simulink library "csc_cac_coarse_acs_cntrl_mtv_lib"  (R2014b)
settings: Solver=ode45  StartTime=0.0  StopTime=10.0  RelTol=1e-3
values from neighbouring files (symbols this model uses):
  attitude_limit = 0.1745    [csu_waypoint_hover_guidance_init.m]
  fsw_dt = 0.1    [csc_est_state_estimation_test.m]    (also in csci_fsw_mtv_init.m)
  kd_attitude = 5.3    [csu_waypoint_hover_guidance_init.m]
  ki_attitude = 15    [csu_waypoint_hover_guidance_init.m]
  kp_attitude = 14.2    [csu_waypoint_hover_guidance_init.m]
  psp_coarse_acs_thrust = 25.5773    [csu_psp_propulstion_system_parameters_mtv_init.m]
  psp_thruster10_orientation = [0.259,0,0.966]    [csu_psp_propulstion_system_parameters_mtv_init.m]
  psp_thruster10_position = [-0.0699,-0.6668,-0.22]    [csu_psp_propulstion_system_parameters_mtv_init.m]
  psp_thruster11_orientation = [0,0,1]    [csu_psp_propulstion_system_parameters_mtv_init.m]
  psp_thruster11_position = [0,-0.6668,-0.22]    [csu_psp_propulstion_system_parameters_mtv_init.m]
  psp_thruster12_orientation = [-0.259,0,0.966]    [csu_psp_propulstion_system_parameters_mtv_init.m]
  psp_thruster12_position = [0.0699,-0.6668,-0.22]    [csu_psp_propulstion_system_parameters_mtv_init.m]
  psp_thruster1_orientation = [0,0.259,0.966]    [csu_psp_propulstion_system_parameters_mtv_init.m]
  psp_thruster1_position = [0.6668,-0.0699,-0.22]    [csu_psp_propulstion_system_parameters_mtv_init.m]
  psp_thruster2_orientation = [0,0,1]    [csu_psp_propulstion_system_parameters_mtv_init.m]
  psp_thruster2_position = [0.6668,0,-0.22]    [csu_psp_propulstion_system_parameters_mtv_init.m]
  psp_thruster3_orientation = [0,-0.259,0.966]    [csu_psp_propulstion_system_parameters_mtv_init.m]
  psp_thruster3_position = [0.6668,0.0699,-0.22]    [csu_psp_propulstion_system_parameters_mtv_init.m]
  psp_thruster4_orientation = [-0.259,0,0.966]    [csu_psp_propulstion_system_parameters_mtv_init.m]
  psp_thruster4_position = [0.0699,0.6668,-0.22]    [csu_psp_propulstion_system_parameters_mtv_init.m]
  psp_thruster5_orientation = [0,0,1]    [csu_psp_propulstion_system_parameters_mtv_init.m]
  psp_thruster5_position = [0,0.6668,-0.22]    [csu_psp_propulstion_system_parameters_mtv_init.m]
  psp_thruster6_orientation = [0.259,0,0.966]    [csu_psp_propulstion_system_parameters_mtv_init.m]
  psp_thruster6_position = [-0.0699,0.6668,-0.22]    [csu_psp_propulstion_system_parameters_mtv_init.m]
  psp_thruster7_orientation = [0,-0.259,0.966]    [csu_psp_propulstion_system_parameters_mtv_init.m]
  psp_thruster7_position = [-0.6668,0.0699,-0.22]    [csu_psp_propulstion_system_parameters_mtv_init.m]
  psp_thruster8_orientation = [0,0,1]    [csu_psp_propulstion_system_parameters_mtv_init.m]
  psp_thruster8_position = [-0.6668,0,-0.22]    [csu_psp_propulstion_system_parameters_mtv_init.m]
  psp_thruster9_orientation = [0,0.259,0.966]    [csu_psp_propulstion_system_parameters_mtv_init.m]
  psp_thruster9_position = [-0.6668,-0.0699,-0.22]    [csu_psp_propulstion_system_parameters_mtv_init.m]
undefined symbols (not defined in the file or in its folder): coarse_thr_on_bias, emp_cgx_location_fillfrac_100, emp_cgy_location_fillfrac_100, emp_cgz_location_fillfrac_100, emp_inertia_wet_dry, emp_mass_wet_dry, force_1_2_3_7_8_9, force_1_to_12, force_2_8, force_4_5_6_10_11_12, force_5_11, Thr2TqF
libraries: simulink x17, vrlib x12, util_quat_lib x2, util_mass_prop_lib x1
settings Model: Creator=tgorton  LastModifiedBy=tgorton

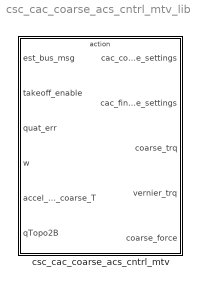
== system csc_cac_coarse_acs_cntrl_mtv_lib ==
  csc_cac_coarse_acs_cntrl_mtv : Subsystem

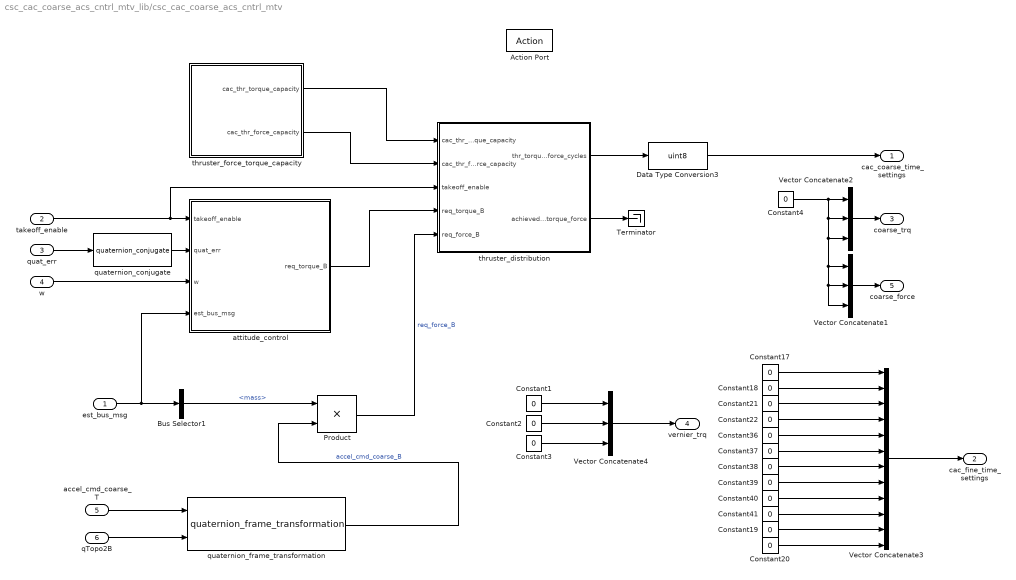
== system csc_cac_coarse_acs_cntrl_mtv_lib/csc_cac_coarse_acs_cntrl_mtv ==
  est_bus_msg : Inport
  takeoff_enable : Inport  Port=2
  quat_err : Inport  Port=3
  w : Inport  Port=4
  accel_cmd_coarse_T : Inport  Port=5
  qTopo2B : Inport  Port=6
  Action Port : ActionPort
  Bus Selector1 : BusSelector  OutputSignals=mass
  Constant{1..4} (4 alike) : Constant  Value=0  OutDataTypeStr=int8
  Constant{17..22,36..41} (12 alike) : Constant  Value=0  OutDataTypeStr=uint8
  Data Type Conversion3 : DataTypeConversion  OutDataTypeStr=uint8
  Product : Product
  Terminator : Terminator
  Vector Concatenate1 : Concatenate  NumInputs=3
  Vector Concatenate2 : Concatenate  NumInputs=3
  Vector Concatenate3 : Concatenate  NumInputs=12
  Vector Concatenate4 : Concatenate  NumInputs=3
  attitude_control : Subsystem
  quaternion_conjugate : util_quat_lib/quaternion_conjugate  SystemSampleTime=-1
  quaternion_frame_transformation : util_quat_lib/quaternion_frame_transformation  SystemSampleTime=-1
  thruster_distribution : Subsystem
  "thruster_force_torque_capacity " : Subsystem
  cac_coarse_time_settings : Outport
  cac_fine_time_settings : Outport  Port=2
  coarse_trq : Outport  Port=3
  vernier_trq : Outport  Port=4
  coarse_force : Outport  Port=5
  wires:
  quaternion_conjugate/1 -> attitude_control/2(quat_err)
  Constant4/1 -> Vector Concatenate2/1, Vector Concatenate2/2, Vector Concatenate2/3, Vector Concatenate1/1, Vector Concatenate1/2, Vector Concatenate1/3
  quaternion_frame_transformation/1 -> Product/2  "accel_cmd_coarse_B"
  accel_cmd_coarse_T/1 -> quaternion_frame_transformation/1
  qTopo2B/1 -> quaternion_frame_transformation/2
  quat_err/1 -> quaternion_conjugate/1
  w/1 -> attitude_control/3(w)
  takeoff_enable/1 -> attitude_control/1(takeoff_enable), thruster_distribution/3(takeoff_enable)
  Vector Concatenate2/1 -> coarse_trq/1
  "thruster_force_torque_capacity "/1(cac_thr_torque_capacity) -> thruster_distribution/1(cac_thr_torque_capacity)
  "thruster_force_torque_capacity "/2(cac_thr_force_capacity) -> thruster_distribution/2(cac_thr_force_capacity)
  attitude_control/1(req_torque_B) -> thruster_distribution/4(req_torque_B)
  Constant17/1 -> Vector Concatenate3/1
  Constant20/1 -> Vector Concatenate3/12
  Constant18/1 -> Vector Concatenate3/2
  Constant19/1 -> Vector Concatenate3/11
  Constant21/1 -> Vector Concatenate3/3
  Constant22/1 -> Vector Concatenate3/4
  Constant41/1 -> Vector Concatenate3/10
  Constant40/1 -> Vector Concatenate3/9
  Constant36/1 -> Vector Concatenate3/5
  Constant37/1 -> Vector Concatenate3/6
  Constant39/1 -> Vector Concatenate3/8
  Constant38/1 -> Vector Concatenate3/7
  Vector Concatenate3/1 -> cac_fine_time_settings/1
  thruster_distribution/1(thr_torque_force_cycles) -> Data Type Conversion3/1
  Vector Concatenate4/1 -> vernier_trq/1
  Constant1/1 -> Vector Concatenate4/1
  Constant2/1 -> Vector Concatenate4/2
  Constant3/1 -> Vector Concatenate4/3
  Data Type Conversion3/1 -> cac_coarse_time_settings/1
  thruster_distribution/2(achieved_torque_force) -> Terminator/1
  Vector Concatenate1/1 -> coarse_force/1
  est_bus_msg/1 -> Bus Selector1/1, attitude_control/4(est_bus_msg)
  Bus Selector1/1 -> Product/1  "<mass>"
  Product/1 -> thruster_distribution/5(req_force_B)  "req_force_B"

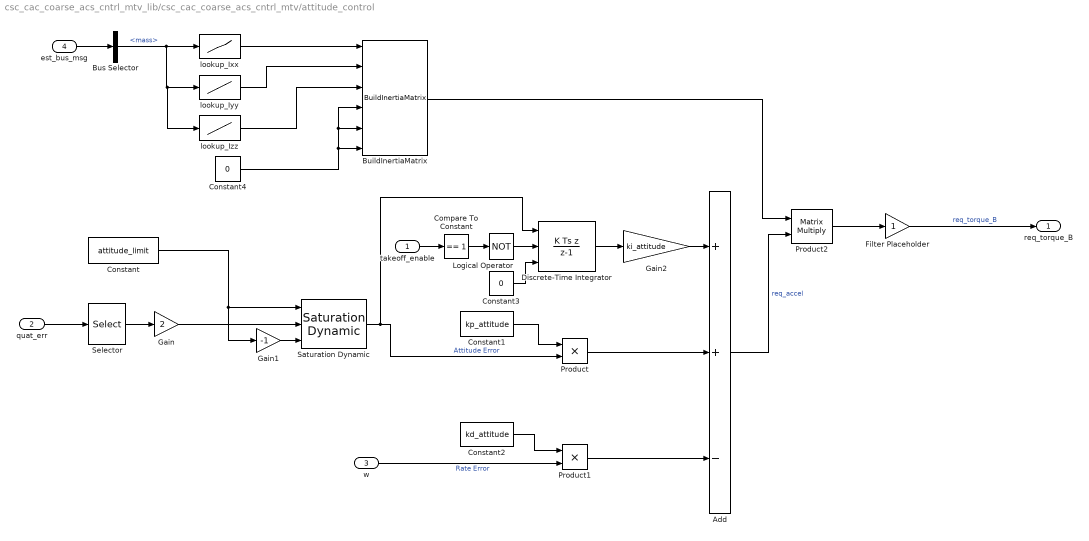
== system csc_cac_coarse_acs_cntrl_mtv_lib/csc_cac_coarse_acs_cntrl_mtv/attitude_control ==
  takeoff_enable : Inport
  quat_err : Inport  Port=2
  w : Inport  Port=3
  est_bus_msg : Inport  Port=4
  Add : Sum  Inputs=++-
  BuildInertiaMatrix : util_mass_prop_lib/BuildInertiaMatrix  SystemSampleTime=-1
  Bus Selector : BusSelector  OutputSignals=mass
  Compare To Constant : simulink/Logic and Bit Operations/Compare To Constant  relop===  const=1  OutDataTypeStr=boolean
  Constant : Constant  Value=attitude_limit
  Constant1 : Constant  Value=kp_attitude
  Constant2 : Constant  Value=kd_attitude
  Constant3 : Constant  Value=0
  Constant4 : Constant  Value=0
  Discrete-Time Integrator : DiscreteIntegrator  IntegratorMethod=Integration: Backward Euler  gainval=1  ExternalReset=level  InitialConditionSource=external  InitialConditionSetting=State (most efficient)  SampleTime=fsw_dt  LimitOutput=on  UpperSaturationLimit=1e6  LowerSaturationLimit=-1e6
  Filter Placeholder : Gain
  Gain : Gain  Gain=2
  Gain1 : Gain  Gain=-1
  Gain2 : Gain  Gain=ki_attitude
  Logical Operator : Logic  Operator=NOT  AllPortsSameDT=off  OutDataTypeStr=boolean
  Product : Product
  Product1 : Product
  Product2 : Product  Multiplication=Matrix(*)
  Saturation Dynamic : simulink/Discontinuities/Saturation Dynamic  OutMin=[]  OutMax=[]  OutDataTypeStr=Inherit: Same as second input  OutDataType=fixdt(1, 16)  OutScaling=2^-10  DoSatur=off
  Selector : Selector  InputPortWidth=4  Indices=[1 2 3]
  lookup_Ixx : Lookup  InputValues=emp_mass_wet_dry  Table=emp_inertia_wet_dry(1,:)
  lookup_Iyy : Lookup  InputValues=emp_mass_wet_dry  Table=emp_inertia_wet_dry(2,:)
  lookup_Izz : Lookup  InputValues=emp_mass_wet_dry  Table=emp_inertia_wet_dry(3,:)
  req_torque_B : Outport
  wires:
  Compare To Constant/1 -> Logical Operator/1
  quat_err/1 -> Selector/1
  Selector/1 -> Gain/1
  Gain/1 -> Saturation Dynamic/2
  Gain1/1 -> Saturation Dynamic/3
  Constant/1 -> Gain1/1, Saturation Dynamic/1
  Saturation Dynamic/1 -> Product/2, Discrete-Time Integrator/1  "Attitude Error"
  w/1 -> Product1/2  "Rate Error"
  Constant1/1 -> Product/1
  Constant2/1 -> Product1/1
  Constant3/1 -> Discrete-Time Integrator/3
  Logical Operator/1 -> Discrete-Time Integrator/2
  takeoff_enable/1 -> Compare To Constant/1
  Discrete-Time Integrator/1 -> Gain2/1
  Product/1 -> Add/2
  Product1/1 -> Add/3
  Add/1 -> Product2/2  "req_accel"
  est_bus_msg/1 -> Bus Selector/1
  Bus Selector/1 -> lookup_Izz/1, lookup_Iyy/1, lookup_Ixx/1  "<mass>"
  lookup_Ixx/1 -> BuildInertiaMatrix/1
  lookup_Iyy/1 -> BuildInertiaMatrix/2
  lookup_Izz/1 -> BuildInertiaMatrix/3
  Constant4/1 -> BuildInertiaMatrix/5, BuildInertiaMatrix/4, BuildInertiaMatrix/6
  BuildInertiaMatrix/1 -> Product2/1
  Product2/1 -> Filter Placeholder/1
  Filter Placeholder/1 -> req_torque_B/1  "req_torque_B"
  Gain2/1 -> Add/1

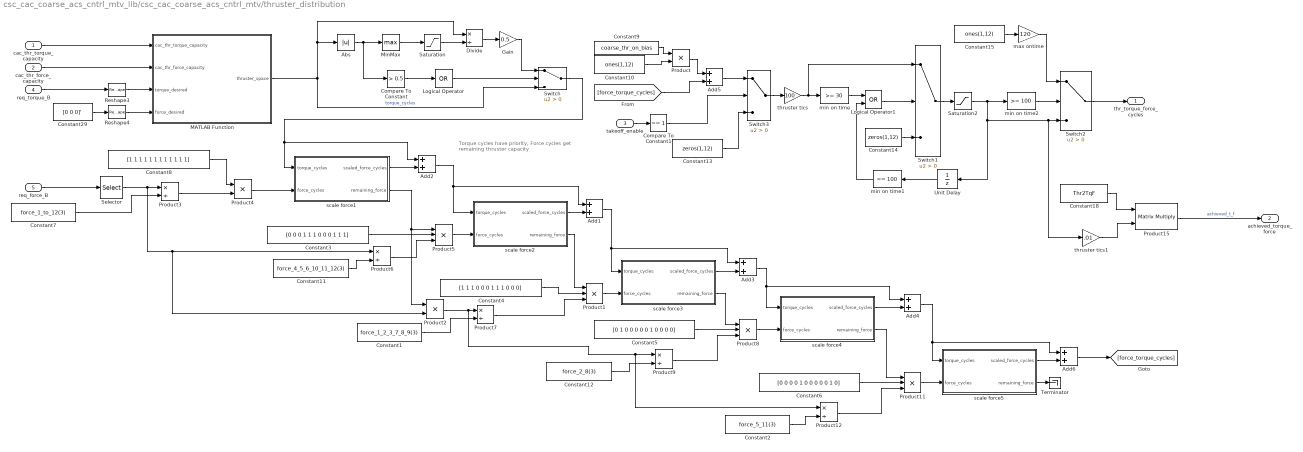
== system csc_cac_coarse_acs_cntrl_mtv_lib/csc_cac_coarse_acs_cntrl_mtv/thruster_distribution ==
  note: Torque cycles have priority, Force cycles
      | get remaining thruster capacity
  cac_thr_torque_capacity : Inport
  cac_thr_force_capacity : Inport  Port=2
  takeoff_enable : Inport  Port=3
  req_torque_B : Inport  Port=4
  req_force_B : Inport  Port=5
  Abs : Abs
  Add{1..6} (6 alike) : Sum
  Compare To Constant : simulink/Logic and Bit Operations/Compare To Constant  relop=>  const=0.5  OutDataTypeStr=boolean
  Compare To Constant1 : simulink/Logic and Bit Operations/Compare To Constant  relop===  const=1  OutDataTypeStr=boolean
  Constant1 : Constant  Value=force_1_2_3_7_8_9(3)
  Constant10 : Constant  Value=ones(1,12)
  Constant11 : Constant  Value=force_4_5_6_10_11_12(3)
  Constant12 : Constant  Value=force_2_8(3)
  Constant13 : Constant  Value=zeros(1,12)
  Constant14 : Constant  Value=zeros(1,12)
  Constant15 : Constant  Value=ones(1,12)
  Constant18 : Constant  Value=Thr2TqF
  Constant2 : Constant  Value=force_5_11(3)
  Constant29 : Constant  Value=[0 0 0]'
  Constant3 : Constant  Value=[0 0 0 1 1 1 0 0 0 1 1 1]
  Constant4 : Constant  Value=[1 1 1 0 0 0 1 1 1 0 0 0]
  Constant5 : Constant  Value=[0 1 0 0 0 0 0 1 0 0 0 0]
  Constant6 : Constant  Value=[0 0 0 0 1 0 0 0 0 0 1 0]
  Constant7 : Constant  Value=force_1_to_12(3)
  Constant8 : Constant  Value=[1 1 1 1 1 1 1 1 1 1 1 1]
  Constant9 : Constant  Value=coarse_thr_on_bias
  Divide : Product  Inputs=*/
  Gain : Gain  Gain=0.5
  Logical Operator : Logic  Operator=OR  Inputs=1  AllPortsSameDT=off  OutDataTypeStr=boolean
  Logical Operator1 : Logic  Operator=OR  AllPortsSameDT=off  OutDataTypeStr=boolean
  MATLAB Function : MATLAB Function  TreatAsAtomicUnit=on
  MinMax : MinMax  Function=max
  Product : Product
  Product{1,5,8,11} (4 alike) : Product  Inputs=3
  Product{3,6..7,9,12} (5 alike) : Product  Inputs=*/
  Product15 : Product  Inputs=**  Multiplication=Matrix(*)
  Product2 : Product  Inputs=**
  Product4 : Product
  Reshape3 : Reshape  OutputDimensionality=Column vector (2-D)
  Reshape4 : Reshape  OutputDimensionality=Column vector (2-D)
  Saturation : Saturate  UpperLimit=1e10  LowerLimit=1e-10
      settings: AttributesFormatString=|
      | %<UpperLimit>
      | %<LowerLimit>
  Saturation2 : Saturate  UpperLimit=100  LowerLimit=0
      settings: AttributesFormatString=|
      | %<UpperLimit>
      | %<LowerLimit>
  Selector : Selector  InputPortWidth=3  Indices=[3]
  Switch{,1..3} (4 alike) : Switch  Criteria=u2 > Threshold
  Terminator : Terminator
  Unit Delay : UnitDelay  SampleTime=-1
  max ontime : Gain  Gain=120
  min on time : simulink/Logic and Bit Operations/Compare To Constant  relop=>=  const=30  OutDataTypeStr=boolean
  min on time1 : simulink/Logic and Bit Operations/Compare To Constant  relop===  const=100  OutDataTypeStr=boolean
  min on time2 : simulink/Logic and Bit Operations/Compare To Constant  relop=>=  const=100  OutDataTypeStr=boolean
  scale force1 : Subsystem
  scale force2 : Subsystem
  scale force3 : Subsystem
  scale force4 : Subsystem
  scale force5 : Subsystem
  thruster tics : Gain  Gain=100
  thruster tics1 : Gain  Gain=.01
  thr_torque_force_cycles : Outport
  achieved_torque_force : Outport  Port=2
  wires:
  Constant13/1 -> Switch3/3
  Switch3/1 -> thruster tics/1
  Compare To Constant1/1 -> Switch3/2
  takeoff_enable/1 -> Compare To Constant1/1
  thruster tics1/1 -> Product15/2
  Product15/1 -> achieved_torque_force/1  "achieved_t_f"
  Constant18/1 -> Product15/1
  Add5/1 -> Switch3/1
  req_torque_B/1 -> Reshape3/1
  Constant29/1 -> Reshape4/1
  Reshape3/1 -> MATLAB Function/3(torque_desired)
  Reshape4/1 -> MATLAB Function/4(force_desired)
  cac_thr_torque_capacity/1 -> MATLAB Function/1(cac_thr_torque_capacity)
  cac_thr_force_capacity/1 -> MATLAB Function/2(cac_thr_force_capacity)
  MinMax/1 -> Saturation/1
  Saturation/1 -> Divide/2
  Compare To Constant/1 -> Logical Operator/1
  Logical Operator/1 -> Switch/2
  Divide/1 -> Gain/1
  Switch/1 -> scale force1/1(torque_cycles), Add2/1
  MATLAB Function/1(thruster_space) -> Abs/1, Divide/1, Switch/3  "torque_cycles"
  Abs/1 -> Compare To Constant/1, MinMax/1
  Gain/1 -> Switch/1
  Add2/1 -> Add1/1, scale force2/1(torque_cycles)
  Selector/1 -> Product2/2, Product6/1, Product3/1
  req_force_B/1 -> Selector/1
  Product3/1 -> Product4/2
  Constant8/1 -> Product4/1
  Constant7/1 -> Product3/2
  Constant3/1 -> Product5/2
  Constant11/1 -> Product6/2
  Product6/1 -> Product5/3
  Product4/1 -> scale force1/2(force_cycles)
  scale force1/1(scaled_force_cycles) -> Add2/2
  scale force1/2(remaining_force) -> Product2/1, Product5/1
  Product5/1 -> scale force2/2(force_cycles)
  scale force2/1(scaled_force_cycles) -> Add1/2
  Add1/1 -> Add3/1, scale force3/1(torque_cycles)
  scale force2/2(remaining_force) -> Product1/1
  Constant1/1 -> Product7/2
  Product2/1 -> Product12/1, Product9/1, Product7/1
  Product7/1 -> Product1/3
  Constant4/1 -> Product1/2
  Product1/1 -> scale force3/2(force_cycles)
  scale force3/1(scaled_force_cycles) -> Add3/2
  Add3/1 -> Add4/1, scale force4/1(torque_cycles)
  scale force3/2(remaining_force) -> Product8/1
  scale force4/2(remaining_force) -> Product11/1
  Product8/1 -> scale force4/2(force_cycles)
  Constant5/1 -> Product8/2
  Product9/1 -> Product8/3
  Constant12/1 -> Product9/2
  scale force4/1(scaled_force_cycles) -> Add4/2
  scale force5/1(scaled_force_cycles) -> Add6/2
  Add4/1 -> Add6/1, scale force5/1(torque_cycles)
  Constant6/1 -> Product11/2
  Product12/1 -> Product11/3
  Constant2/1 -> Product12/2
  Product11/1 -> scale force5/2(force_cycles)
  scale force5/2(remaining_force) -> Terminator/1
  Constant10/1 -> Product/2
  [force_torque_cycles] -> Add5/2
  thruster tics/1 -> Switch1/1, min on time/1
  min on time/1 -> Logical Operator1/1
  Constant14/1 -> Switch1/3
  Switch1/1 -> Saturation2/1
  Saturation2/1 -> min on time2/1, Unit Delay/1, thruster tics1/1, Switch2/3
  Unit Delay/1 -> min on time1/1
  Logical Operator1/1 -> Switch1/2
  min on time1/1 -> Logical Operator1/2
  min on time2/1 -> Switch2/2
  Constant15/1 -> max ontime/1
  max ontime/1 -> Switch2/1
  Switch2/1 -> thr_torque_force_cycles/1
  Add6/1 -> [force_torque_cycles]
  Constant9/1 -> Product/1
  Product/1 -> Add5/1

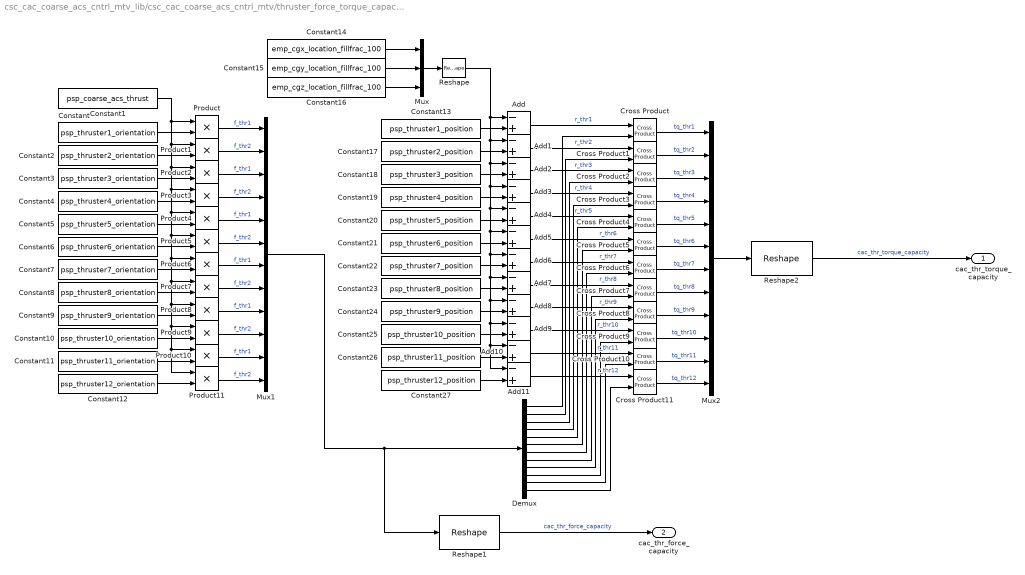
== system csc_cac_coarse_acs_cntrl_mtv_lib/csc_cac_coarse_acs_cntrl_mtv/thruster_force_torque_capacity  ==
  Add{,1..11} (12 alike) : Sum  Inputs=-+
  Constant : Constant  Value=psp_thruster1_orientation
  Constant1 : Constant  Value=psp_coarse_acs_thrust
  Constant10 : Constant  Value=psp_thruster10_orientation
  Constant11 : Constant  Value=psp_thruster11_orientation
  Constant12 : Constant  Value=psp_thruster12_orientation
  Constant13 : Constant  Value=psp_thruster1_position
  Constant14 : Constant  Value=emp_cgx_location_fillfrac_100
  Constant15 : Constant  Value=emp_cgy_location_fillfrac_100
  Constant16 : Constant  Value=emp_cgz_location_fillfrac_100
  Constant17 : Constant  Value=psp_thruster2_position
  Constant18 : Constant  Value=psp_thruster3_position
  Constant19 : Constant  Value=psp_thruster4_position
  Constant2 : Constant  Value=psp_thruster2_orientation
  Constant20 : Constant  Value=psp_thruster5_position
  Constant21 : Constant  Value=psp_thruster6_position
  Constant22 : Constant  Value=psp_thruster7_position
  Constant23 : Constant  Value=psp_thruster8_position
  Constant24 : Constant  Value=psp_thruster9_position
  Constant25 : Constant  Value=psp_thruster10_position
  Constant26 : Constant  Value=psp_thruster11_position
  Constant27 : Constant  Value=psp_thruster12_position
  Constant3 : Constant  Value=psp_thruster3_orientation
  Constant4 : Constant  Value=psp_thruster4_orientation
  Constant5 : Constant  Value=psp_thruster5_orientation
  Constant6 : Constant  Value=psp_thruster6_orientation
  Constant7 : Constant  Value=psp_thruster7_orientation
  Constant8 : Constant  Value=psp_thruster8_orientation
  Constant9 : Constant  Value=psp_thruster9_orientation
  Cross Product{,1..11} (12 alike) : vrlib/Utilities/Cross Product
  Demux : Demux  Outputs=12
  Mux : Mux  Inputs=3
  Mux1 : Mux  Inputs=12
  Mux2 : Mux  Inputs=12
  Product{,1..11} (12 alike) : Product
  Reshape : Reshape  OutputDimensionality=Column vector (2-D)
  Reshape1 : Reshape  OutputDimensionality=Customize  OutputDimensions=[3,12]
  Reshape2 : Reshape  OutputDimensionality=Customize  OutputDimensions=[3,12]
  cac_thr_torque_capacity : Outport
  cac_thr_force_capacity : Outport  Port=2
  wires:
  Constant/1 -> Product/2
  Constant2/1 -> Product1/2
  Product/1 -> Mux1/1  "f_thr1"
  Product1/1 -> Mux1/2  "f_thr2"
  Constant3/1 -> Product2/2
  Constant4/1 -> Product3/2
  Product2/1 -> Mux1/3  "f_thr1"
  Product3/1 -> Mux1/4  "f_thr2"
  Constant5/1 -> Product4/2
  Constant6/1 -> Product5/2
  Product4/1 -> Mux1/5  "f_thr1"
  Product5/1 -> Mux1/6  "f_thr2"
  Constant7/1 -> Product6/2
  Constant8/1 -> Product7/2
  Product6/1 -> Mux1/7  "f_thr1"
  Product7/1 -> Mux1/8  "f_thr2"
  Constant9/1 -> Product8/2
  Constant10/1 -> Product9/2
  Product8/1 -> Mux1/9  "f_thr1"
  Product9/1 -> Mux1/10  "f_thr2"
  Constant11/1 -> Product10/2
  Constant1/1 -> Product2/1, Product4/1, Product6/1, Product8/1, Product10/1, Product11/1, Product9/1, Product7/1, Product5/1, Product3/1, Product1/1, Product/1
  Constant12/1 -> Product11/2
  Product10/1 -> Mux1/11  "f_thr1"
  Product11/1 -> Mux1/12  "f_thr2"
  Constant14/1 -> Mux/1
  Constant15/1 -> Mux/2
  Constant16/1 -> Mux/3
  Mux/1 -> Reshape/1
  Constant13/1 -> Add/2
  Constant17/1 -> Add1/2
  Constant18/1 -> Add2/2
  Constant19/1 -> Add3/2
  Constant20/1 -> Add4/2
  Constant21/1 -> Add5/2
  Constant22/1 -> Add6/2
  Constant23/1 -> Add7/2
  Constant24/1 -> Add8/2
  Reshape/1 -> Add2/1, Add6/1, Add10/1, Add11/1, Add9/1, Add8/1, Add7/1, Add5/1, Add4/1, Add3/1, Add1/1, Add/1
  Constant25/1 -> Add9/2
  Constant26/1 -> Add10/2
  Constant27/1 -> Add11/2
  Mux1/1 -> Reshape1/1, Demux/1
  Add/1 -> Cross Product/1  "r_thr1"
  Demux/1 -> Cross Product/2
  Add1/1 -> Cross Product1/1  "r_thr2"
  Demux/2 -> Cross Product1/2
  Add2/1 -> Cross Product2/1  "r_thr3"
  Add3/1 -> Cross Product3/1  "r_thr4"
  Add4/1 -> Cross Product4/1  "r_thr5"
  Add5/1 -> Cross Product5/1  "r_thr6"
  Add6/1 -> Cross Product6/1  "r_thr7"
  Add7/1 -> Cross Product7/1  "r_thr8"
  Add8/1 -> Cross Product8/1  "r_thr9"
  Add9/1 -> Cross Product9/1  "r_thr10"
  Add10/1 -> Cross Product10/1  "r_thr11"
  Add11/1 -> Cross Product11/1  "r_thr12"
  Demux/3 -> Cross Product2/2
  Demux/4 -> Cross Product3/2
  Demux/5 -> Cross Product4/2
  Demux/6 -> Cross Product5/2
  Demux/7 -> Cross Product6/2
  Demux/8 -> Cross Product7/2
  Demux/9 -> Cross Product8/2
  Demux/10 -> Cross Product9/2
  Demux/11 -> Cross Product10/2
  Demux/12 -> Cross Product11/2
  Reshape1/1 -> cac_thr_force_capacity/1  "cac_thr_force_capacity"
  Cross Product/1 -> Mux2/1  "tq_thr1"
  Cross Product1/1 -> Mux2/2  "tq_thr2"
  Cross Product2/1 -> Mux2/3  "tq_thr3"
  Cross Product3/1 -> Mux2/4  "tq_thr4"
  Cross Product4/1 -> Mux2/5  "tq_thr5"
  Cross Product5/1 -> Mux2/6  "tq_thr6"
  Cross Product7/1 -> Mux2/8  "tq_thr8"
  Cross Product6/1 -> Mux2/7  "tq_thr7"
  Cross Product8/1 -> Mux2/9  "tq_thr9"
  Cross Product9/1 -> Mux2/10  "tq_thr10"
  Cross Product10/1 -> Mux2/11  "tq_thr11"
  Cross Product11/1 -> Mux2/12  "tq_thr12"
  Mux2/1 -> Reshape2/1
  Reshape2/1 -> cac_thr_torque_capacity/1  "cac_thr_torque_capacity"

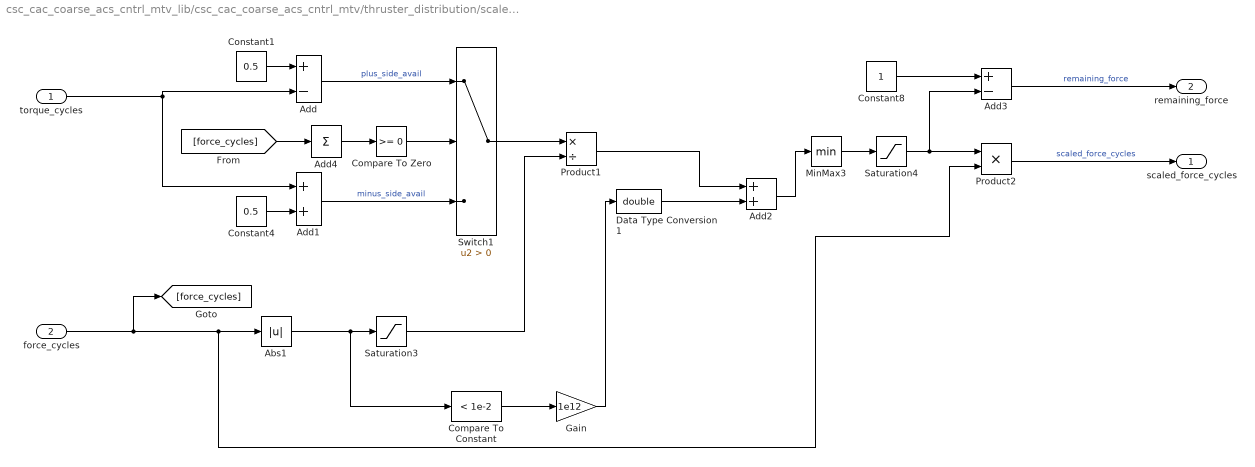
== system csc_cac_coarse_acs_cntrl_mtv_lib/csc_cac_coarse_acs_cntrl_mtv/thruster_distribution/scale force1 ==
  torque_cycles : Inport
  force_cycles : Inport  Port=2
  Abs1 : Abs
  Add : Sum  Inputs=+-
  Add1 : Sum
  Add2 : Sum  InputSameDT=on
  Add3 : Sum  Inputs=+-
  Add4 : Sum  Inputs=+
  Compare To Constant : simulink/Logic and Bit Operations/Compare To Constant  relop=<  const=1e-2  OutDataTypeStr=boolean
  Compare To Zero : simulink/Logic and Bit Operations/Compare To Zero  relop=>=  OutDataTypeStr=boolean
  Constant1 : Constant  Value=0.5
  Constant4 : Constant  Value=0.5
  Constant8 : Constant
  Data Type Conversion1 : DataTypeConversion  OutDataTypeStr=double
  Gain : Gain  Gain=1e12
  MinMax3 : MinMax
  Product1 : Product  Inputs=*/
  Product2 : Product
  Saturation3 : Saturate  UpperLimit=1e10  LowerLimit=1e-10
      settings: AttributesFormatString=|
      | %<UpperLimit>
      | %<LowerLimit>
  Saturation4 : Saturate  UpperLimit=1  LowerLimit=0
      settings: AttributesFormatString=|
      | %<UpperLimit>
      | %<LowerLimit>
  Switch1 : Switch  Criteria=u2 > Threshold
  scaled_force_cycles : Outport
  remaining_force : Outport  Port=2
  wires:
  [force_cycles] -> Add4/1
  Add2/1 -> MinMax3/1
  Gain/1 -> Data Type Conversion1/1
  Compare To Constant/1 -> Gain/1
  Saturation3/1 -> Product1/2
  Saturation4/1 -> Add3/2, Product2/1
  Switch1/1 -> Product1/1
  Product1/1 -> Add2/1
  torque_cycles/1 -> Add/2, Add1/1
  Add3/1 -> remaining_force/1  "remaining_force"
  Add/1 -> Switch1/1  "plus_side_avail"
  Constant1/1 -> Add/1
  Product2/1 -> scaled_force_cycles/1  "scaled_force_cycles"
  force_cycles/1 -> [force_cycles], Product2/2, Abs1/1
  Constant4/1 -> Add1/2
  Add1/1 -> Switch1/3  "minus_side_avail"
  Constant8/1 -> Add3/1
  Compare To Zero/1 -> Switch1/2
  Add4/1 -> Compare To Zero/1
  MinMax3/1 -> Saturation4/1
  Abs1/1 -> Saturation3/1, Compare To Constant/1
  Data Type Conversion1/1 -> Add2/2

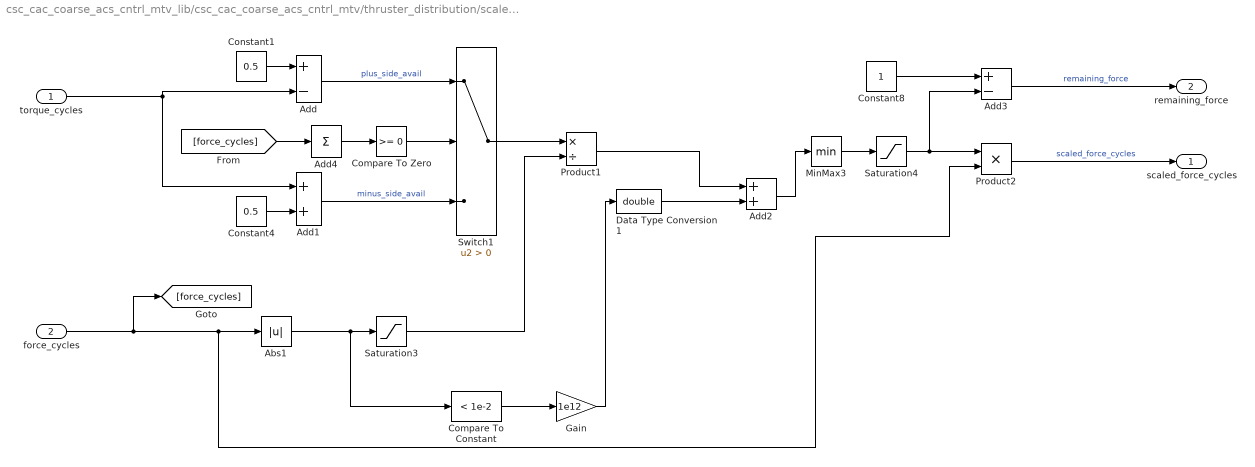
== system csc_cac_coarse_acs_cntrl_mtv_lib/csc_cac_coarse_acs_cntrl_mtv/thruster_distribution/scale force2 ==
  torque_cycles : Inport
  force_cycles : Inport  Port=2
  Abs1 : Abs
  Add : Sum  Inputs=+-
  Add1 : Sum
  Add2 : Sum  InputSameDT=on
  Add3 : Sum  Inputs=+-
  Add4 : Sum  Inputs=+
  Compare To Constant : simulink/Logic and Bit Operations/Compare To Constant  relop=<  const=1e-2  OutDataTypeStr=boolean
  Compare To Zero : simulink/Logic and Bit Operations/Compare To Zero  relop=>=  OutDataTypeStr=boolean
  Constant1 : Constant  Value=0.5
  Constant4 : Constant  Value=0.5
  Constant8 : Constant
  Data Type Conversion1 : DataTypeConversion  OutDataTypeStr=double
  Gain : Gain  Gain=1e12
  MinMax3 : MinMax
  Product1 : Product  Inputs=*/
  Product2 : Product
  Saturation3 : Saturate  UpperLimit=1e10  LowerLimit=1e-10
      settings: AttributesFormatString=|
      | %<UpperLimit>
      | %<LowerLimit>
  Saturation4 : Saturate  UpperLimit=1  LowerLimit=0
      settings: AttributesFormatString=|
      | %<UpperLimit>
      | %<LowerLimit>
  Switch1 : Switch  Criteria=u2 > Threshold
  scaled_force_cycles : Outport
  remaining_force : Outport  Port=2
  wires:
  Data Type Conversion1/1 -> Add2/2
  Abs1/1 -> Compare To Constant/1, Saturation3/1
  MinMax3/1 -> Saturation4/1
  Add4/1 -> Compare To Zero/1
  Compare To Zero/1 -> Switch1/2
  Constant8/1 -> Add3/1
  Add1/1 -> Switch1/3  "minus_side_avail"
  Constant4/1 -> Add1/2
  force_cycles/1 -> Abs1/1, Product2/2, [force_cycles]
  Product2/1 -> scaled_force_cycles/1  "scaled_force_cycles"
  Constant1/1 -> Add/1
  Add/1 -> Switch1/1  "plus_side_avail"
  Add3/1 -> remaining_force/1  "remaining_force"
  torque_cycles/1 -> Add1/1, Add/2
  Product1/1 -> Add2/1
  Switch1/1 -> Product1/1
  Saturation4/1 -> Product2/1, Add3/2
  Saturation3/1 -> Product1/2
  Compare To Constant/1 -> Gain/1
  Gain/1 -> Data Type Conversion1/1
  Add2/1 -> MinMax3/1
  [force_cycles] -> Add4/1

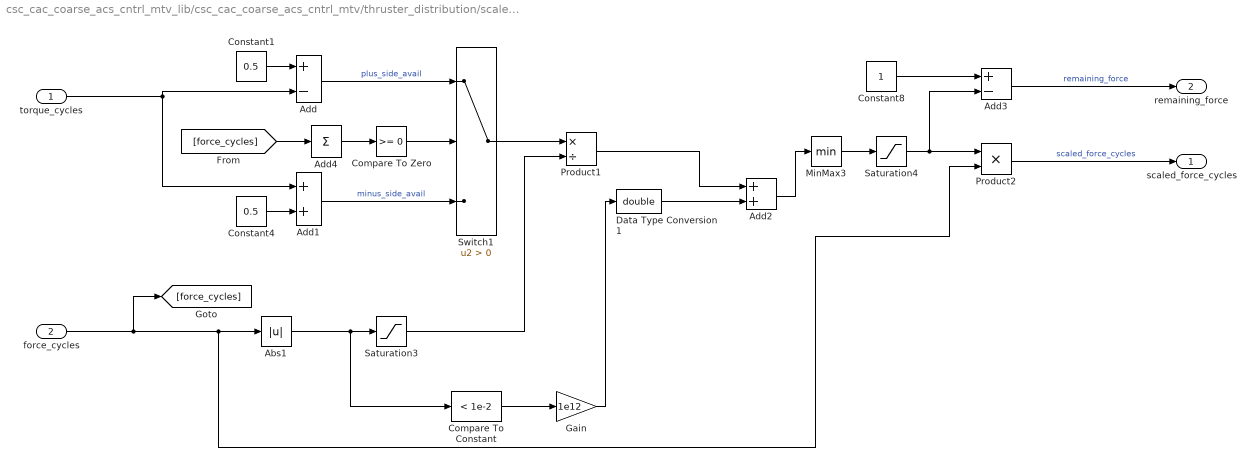
== system csc_cac_coarse_acs_cntrl_mtv_lib/csc_cac_coarse_acs_cntrl_mtv/thruster_distribution/scale force3 ==
  torque_cycles : Inport
  force_cycles : Inport  Port=2
  Abs1 : Abs
  Add : Sum  Inputs=+-
  Add1 : Sum
  Add2 : Sum  InputSameDT=on
  Add3 : Sum  Inputs=+-
  Add4 : Sum  Inputs=+
  Compare To Constant : simulink/Logic and Bit Operations/Compare To Constant  relop=<  const=1e-2  OutDataTypeStr=boolean
  Compare To Zero : simulink/Logic and Bit Operations/Compare To Zero  relop=>=  OutDataTypeStr=boolean
  Constant1 : Constant  Value=0.5
  Constant4 : Constant  Value=0.5
  Constant8 : Constant
  Data Type Conversion1 : DataTypeConversion  OutDataTypeStr=double
  Gain : Gain  Gain=1e12
  MinMax3 : MinMax
  Product1 : Product  Inputs=*/
  Product2 : Product
  Saturation3 : Saturate  UpperLimit=1e10  LowerLimit=1e-10
      settings: AttributesFormatString=|
      | %<UpperLimit>
      | %<LowerLimit>
  Saturation4 : Saturate  UpperLimit=1  LowerLimit=0
      settings: AttributesFormatString=|
      | %<UpperLimit>
      | %<LowerLimit>
  Switch1 : Switch  Criteria=u2 > Threshold
  scaled_force_cycles : Outport
  remaining_force : Outport  Port=2
  wires:
  [force_cycles] -> Add4/1
  Add2/1 -> MinMax3/1
  Gain/1 -> Data Type Conversion1/1
  Compare To Constant/1 -> Gain/1
  Saturation3/1 -> Product1/2
  Saturation4/1 -> Add3/2, Product2/1
  Switch1/1 -> Product1/1
  Product1/1 -> Add2/1
  torque_cycles/1 -> Add/2, Add1/1
  Add3/1 -> remaining_force/1  "remaining_force"
  Add/1 -> Switch1/1  "plus_side_avail"
  Constant1/1 -> Add/1
  Product2/1 -> scaled_force_cycles/1  "scaled_force_cycles"
  force_cycles/1 -> [force_cycles], Product2/2, Abs1/1
  Constant4/1 -> Add1/2
  Add1/1 -> Switch1/3  "minus_side_avail"
  Constant8/1 -> Add3/1
  Compare To Zero/1 -> Switch1/2
  Add4/1 -> Compare To Zero/1
  MinMax3/1 -> Saturation4/1
  Abs1/1 -> Saturation3/1, Compare To Constant/1
  Data Type Conversion1/1 -> Add2/2

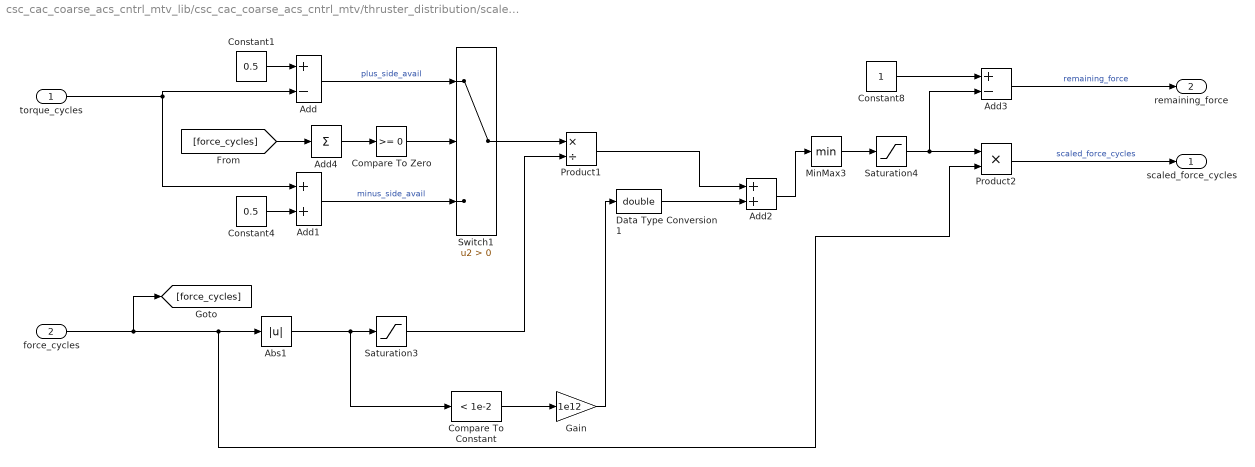
== system csc_cac_coarse_acs_cntrl_mtv_lib/csc_cac_coarse_acs_cntrl_mtv/thruster_distribution/scale force4 ==
  torque_cycles : Inport
  force_cycles : Inport  Port=2
  Abs1 : Abs
  Add : Sum  Inputs=+-
  Add1 : Sum
  Add2 : Sum  InputSameDT=on
  Add3 : Sum  Inputs=+-
  Add4 : Sum  Inputs=+
  Compare To Constant : simulink/Logic and Bit Operations/Compare To Constant  relop=<  const=1e-2  OutDataTypeStr=boolean
  Compare To Zero : simulink/Logic and Bit Operations/Compare To Zero  relop=>=  OutDataTypeStr=boolean
  Constant1 : Constant  Value=0.5
  Constant4 : Constant  Value=0.5
  Constant8 : Constant
  Data Type Conversion1 : DataTypeConversion  OutDataTypeStr=double
  Gain : Gain  Gain=1e12
  MinMax3 : MinMax
  Product1 : Product  Inputs=*/
  Product2 : Product
  Saturation3 : Saturate  UpperLimit=1e10  LowerLimit=1e-10
      settings: AttributesFormatString=|
      | %<UpperLimit>
      | %<LowerLimit>
  Saturation4 : Saturate  UpperLimit=1  LowerLimit=0
      settings: AttributesFormatString=|
      | %<UpperLimit>
      | %<LowerLimit>
  Switch1 : Switch  Criteria=u2 > Threshold
  scaled_force_cycles : Outport
  remaining_force : Outport  Port=2
  wires:
  Data Type Conversion1/1 -> Add2/2
  Abs1/1 -> Compare To Constant/1, Saturation3/1
  MinMax3/1 -> Saturation4/1
  Add4/1 -> Compare To Zero/1
  Compare To Zero/1 -> Switch1/2
  Constant8/1 -> Add3/1
  Add1/1 -> Switch1/3  "minus_side_avail"
  Constant4/1 -> Add1/2
  force_cycles/1 -> Abs1/1, Product2/2, [force_cycles]
  Product2/1 -> scaled_force_cycles/1  "scaled_force_cycles"
  Constant1/1 -> Add/1
  Add/1 -> Switch1/1  "plus_side_avail"
  Add3/1 -> remaining_force/1  "remaining_force"
  torque_cycles/1 -> Add1/1, Add/2
  Product1/1 -> Add2/1
  Switch1/1 -> Product1/1
  Saturation4/1 -> Product2/1, Add3/2
  Saturation3/1 -> Product1/2
  Compare To Constant/1 -> Gain/1
  Gain/1 -> Data Type Conversion1/1
  Add2/1 -> MinMax3/1
  [force_cycles] -> Add4/1

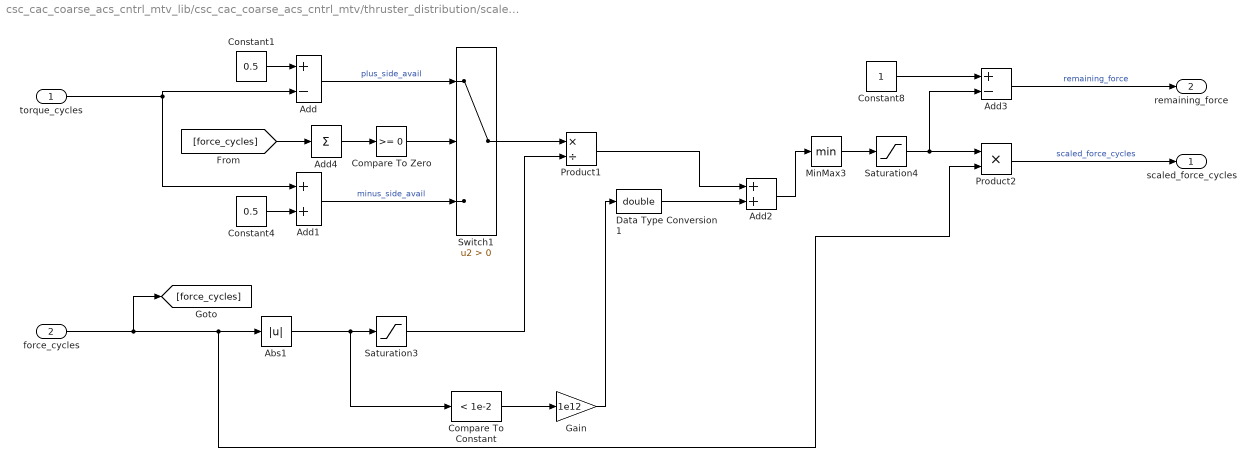
== system csc_cac_coarse_acs_cntrl_mtv_lib/csc_cac_coarse_acs_cntrl_mtv/thruster_distribution/scale force5 ==
  torque_cycles : Inport
  force_cycles : Inport  Port=2
  Abs1 : Abs
  Add : Sum  Inputs=+-
  Add1 : Sum
  Add2 : Sum  InputSameDT=on
  Add3 : Sum  Inputs=+-
  Add4 : Sum  Inputs=+
  Compare To Constant : simulink/Logic and Bit Operations/Compare To Constant  relop=<  const=1e-2  OutDataTypeStr=boolean
  Compare To Zero : simulink/Logic and Bit Operations/Compare To Zero  relop=>=  OutDataTypeStr=boolean
  Constant1 : Constant  Value=0.5
  Constant4 : Constant  Value=0.5
  Constant8 : Constant
  Data Type Conversion1 : DataTypeConversion  OutDataTypeStr=double
  Gain : Gain  Gain=1e12
  MinMax3 : MinMax
  Product1 : Product  Inputs=*/
  Product2 : Product
  Saturation3 : Saturate  UpperLimit=1e10  LowerLimit=1e-10
      settings: AttributesFormatString=|
      | %<UpperLimit>
      | %<LowerLimit>
  Saturation4 : Saturate  UpperLimit=1  LowerLimit=0
      settings: AttributesFormatString=|
      | %<UpperLimit>
      | %<LowerLimit>
  Switch1 : Switch  Criteria=u2 > Threshold
  scaled_force_cycles : Outport
  remaining_force : Outport  Port=2
  wires:
  [force_cycles] -> Add4/1
  Add2/1 -> MinMax3/1
  Gain/1 -> Data Type Conversion1/1
  Compare To Constant/1 -> Gain/1
  Saturation3/1 -> Product1/2
  Saturation4/1 -> Add3/2, Product2/1
  Switch1/1 -> Product1/1
  Product1/1 -> Add2/1
  torque_cycles/1 -> Add/2, Add1/1
  Add3/1 -> remaining_force/1  "remaining_force"
  Add/1 -> Switch1/1  "plus_side_avail"
  Constant1/1 -> Add/1
  Product2/1 -> scaled_force_cycles/1  "scaled_force_cycles"
  force_cycles/1 -> [force_cycles], Product2/2, Abs1/1
  Constant4/1 -> Add1/2
  Add1/1 -> Switch1/3  "minus_side_avail"
  Constant8/1 -> Add3/1
  Compare To Zero/1 -> Switch1/2
  Add4/1 -> Compare To Zero/1
  MinMax3/1 -> Saturation4/1
  Abs1/1 -> Saturation3/1, Compare To Constant/1
  Data Type Conversion1/1 -> Add2/2

== matlab function csc_cac_coarse_acs_cntrl_mtv_lib/csc_cac_coarse_acs_cntrl_mtv/thruster_distribution/MATLAB Function ==
  data: cac_thr_torque_capacity input; thruster_space output; cac_thr_force_capacity input; torque_desired input; force_desired input
function thruster_space = fcn(cac_thr_torque_capacity,cac_thr_force_capacity,torque_desired,force_desired)
%#codegen

thruster_to_torque_and_force = [cac_thr_torque_capacity;
                                cac_thr_force_capacity];
                            
torque_and_force_to_thruster = pinv(thruster_to_torque_and_force);

thruster_space = torque_and_force_to_thruster * [torque_desired; force_desired];
